simulink model "drone_diagram"  (R2021a)
settings: Solver=VariableStepAuto  StartTime=0.0  StopTime=10.0  RelTol=1e-3
values from neighbouring files (symbols this model uses):
  air_density = 1.225    [param_set.m]
  g = 9.8    [param_set.m]
  J = [Jxx 0 0; 0 Jyy 0; 0 0 Jzz]    [linearize_lqr.m]    (also in param_set.m)
  m = 1.5    [param_set.m]
  mixer_matrix = inv(dynamics_matrix)    [param_set.m]
  motor_mix_vector = [1 -1 1 -1]    [param_set.m]
  set_points = [1 0 hover_height 0 0 0 0 0 0 0 0 0]'    [linearize_lqr.m]    (also in param_set.m)
undefined symbols (not defined in the file or in its folder): c_p, lqr_K, lumped_matrix, m_b_a, motor_n_eq, offset, prop_diam, prop_j, slope, x_dist, y_dist
libraries: vrlib x3, aerolibutil x1, dspmtrx3 x1
settings Model: Creator=willwu  LastModifiedBy=Willi

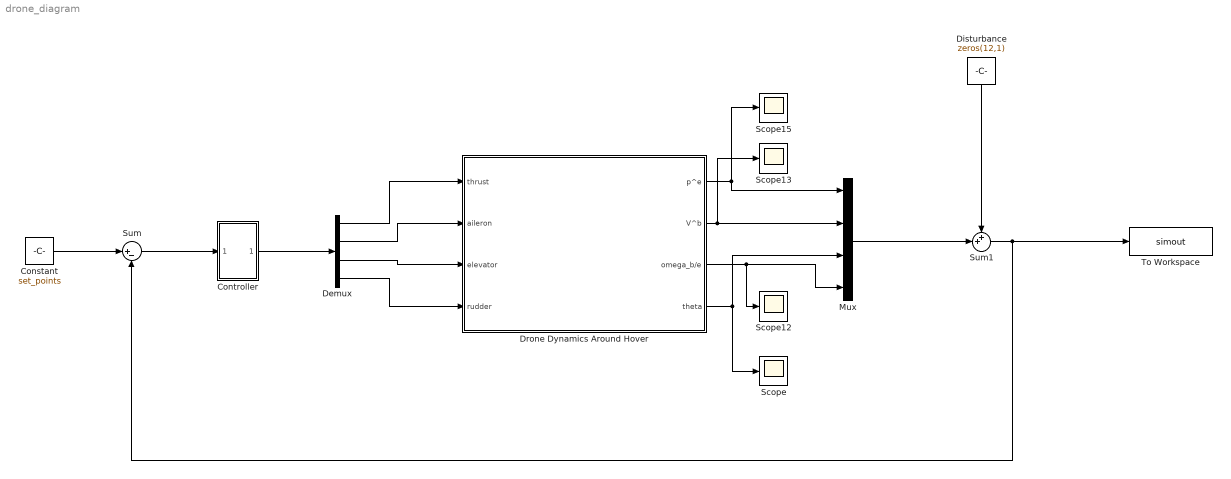
== system drone_diagram ==
  Constant : Constant  Value=set_points
  Controller : Subsystem
  Demux : Demux
  Disturbance : Constant  Value=zeros(12,1)
  Drone Dynamics Around Hover : Subsystem
  Mux : Mux
  Scope{,12..13,15} (4 alike) : Scope
  Sum : Sum  Inputs=|+-
  Sum1 : Sum  Inputs=++|
  To Workspace : ToWorkspace  VariableName=simout  SaveFormat=Timeseries  SampleTime=-1
  wires:
  Drone Dynamics Around Hover/1(p^e) -> Scope15/1, Mux/1
  Drone Dynamics Around Hover/2(V^b) -> Mux/2, Scope13/1
  Drone Dynamics Around Hover/3(omega_b/e) -> Mux/4, Scope12/1
  Drone Dynamics Around Hover/4(theta) -> Scope/1, Mux/3
  Demux/1 -> Drone Dynamics Around Hover/1(thrust)
  Demux/2 -> Drone Dynamics Around Hover/2(aileron)
  Demux/3 -> Drone Dynamics Around Hover/3(elevator)
  Demux/4 -> Drone Dynamics Around Hover/4(rudder)
  Constant/1 -> Sum/1
  Sum/1 -> Controller/1(In1)
  Controller/1(Out1) -> Demux/1
  Mux/1 -> Sum1/2
  Sum1/1 -> Sum/2, To Workspace/1
  Disturbance/1 -> Sum1/1

== system drone_diagram/Controller ==
  In1 : Inport
  Gain : Gain  Gain=lqr_K  Multiplication=Matrix(K*u)
  Out1 : Outport
  wires:
  In1/1 -> Gain/1
  Gain/1 -> Out1/1

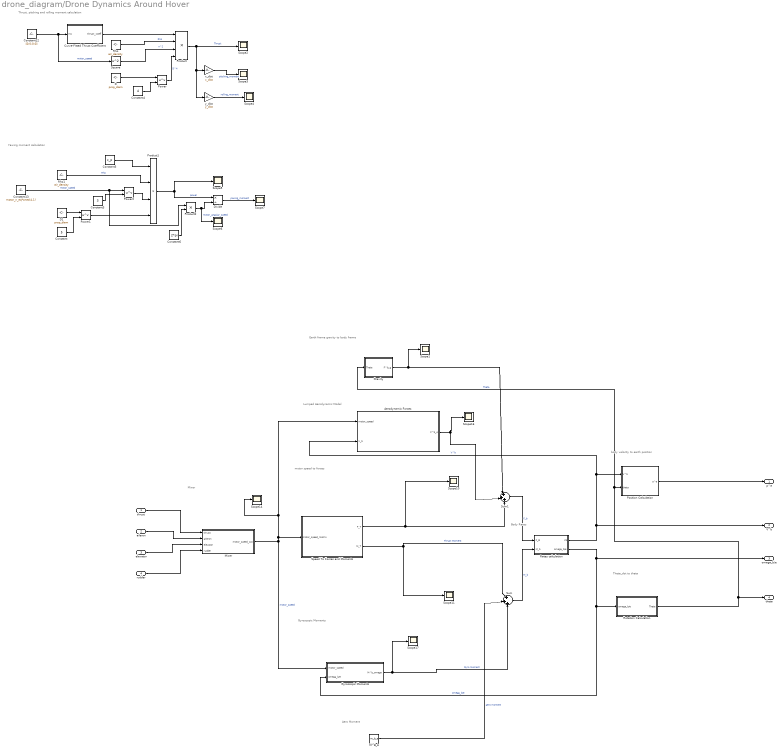
== system drone_diagram/Drone Dynamics Around Hover ==
  note: Aero Moment
  note: Mixer
  note: Gyroscopic Moments
  note: Lumped Aerodynamic Model
  note: body velocity to earth position
  note: motor speed to forces
  note: Earth frame gravity to body frame
  note: Theta_dot to theta
  note: Body Rates
  note: Yawing moment calculation
  note: Thrust, pitching and rolling moment calculation
  thrust : Inport
  aileron : Inport  Port=2
  elevator : Inport  Port=3
  rudder : Inport  Port=4
  Aerodynamic Forces : Subsystem
  Constant : Constant  Value=5
  Constant12 : Constant  Value=[0;0;0;0]
  Constant13 : Constant  Value=motor_n_eq*ones(4,1)
  Constant3 : Constant  Value=3
  Constant4 : Constant  Value=4
  Constant5 : Constant  Value=c_p
  Constant6 : Constant  Value=2*pi
  Curve-Fitted Thrust Coefficient : Subsystem
  D : Constant  Value=prop_diam
  D1 : Constant  Value=prop_diam
  Divide : Product  Inputs=*/
  Gravity : Subsystem
  Gyroscopic Moments : Subsystem
  M^B_A : Constant  Value=m_b_a
  Mixer : Subsystem
  Position Calculation : Subsystem
  Power : Math  Operator=pow  SaturateOnIntegerOverflow=on
  Power1 : Math  Operator=pow  SaturateOnIntegerOverflow=on
  Power2 : Math  Operator=pow  SaturateOnIntegerOverflow=on
  Product : Product  Inputs=4
  Product1 : Product  Inputs=4
  Product2 : Product
  Rates calculation : Subsystem
  Rho : Constant  Value=air_density
  Rho1 : Constant  Value=air_density
  Rotation Calculation : Subsystem
  Scope{1..7,10..11,14,16..17} (12 alike) : Scope
  Speed To Forces and Moments : Subsystem
  Square : Math  Operator=square  SaturateOnIntegerOverflow=on
  Sum : Sum  Inputs=|+|+|+
  Sum1 : Sum  Inputs=|+|+|+
  x_dist : Gain  Gain=x_dist
  y_dist : Gain  Gain=y_dist
  p^e : Outport
  V^b : Outport  Port=2
  omega_b/e : Outport  Port=3
  theta : Outport  Port=4
  wires:
  Sum1/1 -> Rates calculation/1(F_B)  "F_b"
  Aerodynamic Forces/1(F^b_A) -> Scope16/1, Sum1/2
  Mixer/1(motor_speed_out) -> Speed To Forces and Moments/1(motor_speed_matrix), Aerodynamic Forces/1(motor_speed), Scope14/1, Gyroscopic Moments/1(motor_speed)  "motor_speed"
  Sum/1 -> Rates calculation/2(M_b)  "M_b"
  Rotation Calculation/1(Theta) -> theta/1, Gravity/1(Theta), Position Calculation/2(theta)  "Theta"
  Rates calculation/2(omega_b/e) -> omega_b/e/1, Gyroscopic Moments/2(omega_b/e), Rotation Calculation/1(omega_b/e)  "omega_b/e"
  Speed To Forces and Moments/2(M_T) -> Sum/1, Scope11/1  "Thrust Moment"
  Gravity/1(F^b_g) -> Sum1/1, Scope1/1
  Rates calculation/1(Vb) -> V^b/1, Aerodynamic Forces/2(V_b), Position Calculation/1(V^b)  "V^b"
  Gyroscopic Moments/1(M^b_omega) -> Sum/3, Scope17/1  "Gyro moment"
  Speed To Forces and Moments/1(F_T) -> Sum1/3, Scope10/1
  M^B_A/1 -> Sum/2  "aero moment"
  Position Calculation/1(p^e) -> p^e/1
  elevator/1 -> Mixer/3(elevator)
  thrust/1 -> Mixer/1(thrust)
  aileron/1 -> Mixer/2(aileron)
  rudder/1 -> Mixer/4(rudder)
  y_dist/1 -> Scope4/1  "rolling_moment"
  Constant6/1 -> Product2/2
  Product1/1 -> Scope5/1, Divide/1  "power"
  Rho1/1 -> Product1/2  "Rho"
  Constant12/1 -> Square/1, Curve-Fitted Thrust Coefficient/1(In1)  "motor_speed"
  Power1/1 -> Product1/4
  Constant3/1 -> Power2/2
  Constant/1 -> Power1/2
  Power2/1 -> Product1/3
  D1/1 -> Power1/1
  Power/1 -> Product/4  "D^4"
  Product2/1 -> Scope6/1, Divide/2  "motor_angular_speed"
  Square/1 -> Product/3  "n^2"
  Product/1 -> Scope2/1, y_dist/1, x_dist/1  "Thrust"
  Rho/1 -> Product/2  "Rho"
  Constant4/1 -> Power/2
  Divide/1 -> Scope7/1  "yawing_moment"
  Constant5/1 -> Product1/1
  Constant13/1 -> Product2/1, Power2/1  "Motor_speed"
  x_dist/1 -> Scope3/1  "pitching_moment"
  D/1 -> Power/1
  Curve-Fitted Thrust Coefficient/1(thrust_coeff) -> Product/1

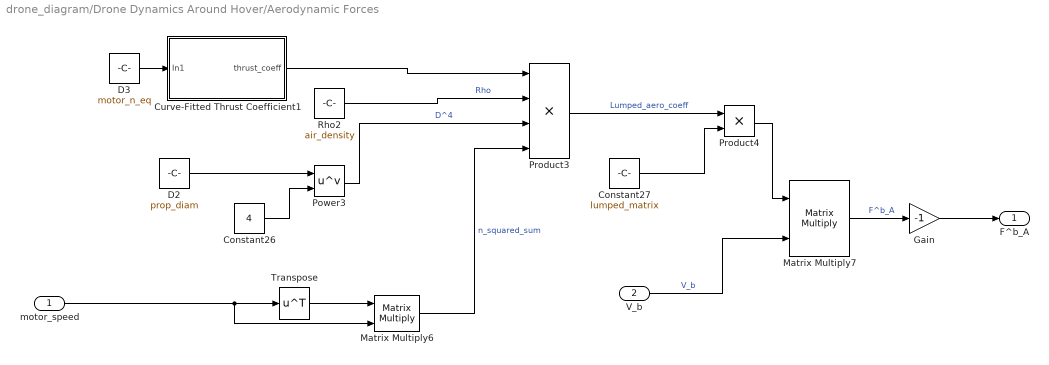
== system drone_diagram/Drone Dynamics Around Hover/Aerodynamic Forces ==
  motor_speed : Inport
  V_b : Inport  Port=2
  Constant26 : Constant  Value=4
  Constant27 : Constant  Value=lumped_matrix
  Curve-Fitted Thrust Coefficient1 : Subsystem
  D2 : Constant  Value=prop_diam
  D3 : Constant  Value=motor_n_eq
  Gain : Gain  Gain=-1
  Matrix Multiply6 : Product  Multiplication=Matrix(*)
  Matrix Multiply7 : Product  Multiplication=Matrix(*)
  Power3 : Math  Operator=pow  SaturateOnIntegerOverflow=on
  Product3 : Product  Inputs=4
  Product4 : Product
  Rho2 : Constant  Value=air_density
  Transpose : Math  Operator=transpose  SaturateOnIntegerOverflow=on
  F^b_A : Outport
  wires:
  V_b/1 -> Matrix Multiply7/2  "V_b"
  Matrix Multiply6/1 -> Product3/4  "n_squared_sum"
  Power3/1 -> Product3/3  "D^4"
  D3/1 -> Curve-Fitted Thrust Coefficient1/1(In1)
  Constant27/1 -> Product4/2
  Rho2/1 -> Product3/2  "Rho"
  Product3/1 -> Product4/1  "Lumped_aero_coeff"
  motor_speed/1 -> Matrix Multiply6/2, Transpose/1
  Product4/1 -> Matrix Multiply7/1
  Transpose/1 -> Matrix Multiply6/1
  Constant26/1 -> Power3/2
  D2/1 -> Power3/1
  Curve-Fitted Thrust Coefficient1/1(thrust_coeff) -> Product3/1
  Matrix Multiply7/1 -> Gain/1  "F^b_A"
  Gain/1 -> F^b_A/1

== system drone_diagram/Drone Dynamics Around Hover/Curve-Fitted Thrust Coefficient ==
  In1 : Inport
  Constant : Constant  Value=offset
  Gain2 : Gain  Gain=slope
  Sum2 : Sum  Inputs=|++
  thrust_coeff : Outport
  wires:
  Constant/1 -> Sum2/2  "offset"
  Gain2/1 -> Sum2/1  "slope * n"
  Sum2/1 -> thrust_coeff/1  "thrust_coeff"
  In1/1 -> Gain2/1

== system drone_diagram/Drone Dynamics Around Hover/Gravity ==
  Theta : Inport
  Constant11 : Constant  Value=[0;0;-m*g]
  Matrix Multiply3 : Product  Multiplication=Matrix(*)
  theta_2_rotate E->b : MATLAB Function  TreatAsAtomicUnit=on
  F^b_g : Outport
  wires:
  theta_2_rotate E->b/1(y) -> Matrix Multiply3/1  "RE->b"
  Constant11/1 -> Matrix Multiply3/2  "F^e_g"
  Matrix Multiply3/1 -> F^b_g/1  "F^b_g"
  Theta/1 -> theta_2_rotate E->b/1(u)

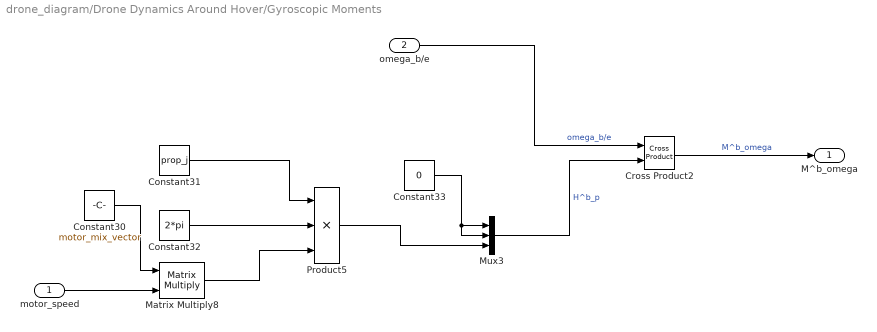
== system drone_diagram/Drone Dynamics Around Hover/Gyroscopic Moments ==
  motor_speed : Inport
  omega_b/e : Inport  Port=2
  Constant30 : Constant  Value=motor_mix_vector  VectorParams1D=off
  Constant31 : Constant  Value=prop_j
  Constant32 : Constant  Value=2*pi
  Constant33 : Constant  Value=0
  Cross Product2 : vrlib/Utilities/Cross Product
  Matrix Multiply8 : Product  Multiplication=Matrix(*)
  Mux3 : Mux  Inputs=3
  Product5 : Product  Inputs=3
  M^b_omega : Outport
  wires:
  Constant30/1 -> Matrix Multiply8/1
  Constant33/1 -> Mux3/2, Mux3/1
  Matrix Multiply8/1 -> Product5/3
  Constant32/1 -> Product5/2
  Product5/1 -> Mux3/3
  omega_b/e/1 -> Cross Product2/1  "omega_b/e"
  Constant31/1 -> Product5/1
  Mux3/1 -> Cross Product2/2  "H^b_p"
  motor_speed/1 -> Matrix Multiply8/2
  Cross Product2/1 -> M^b_omega/1  "M^b_omega"

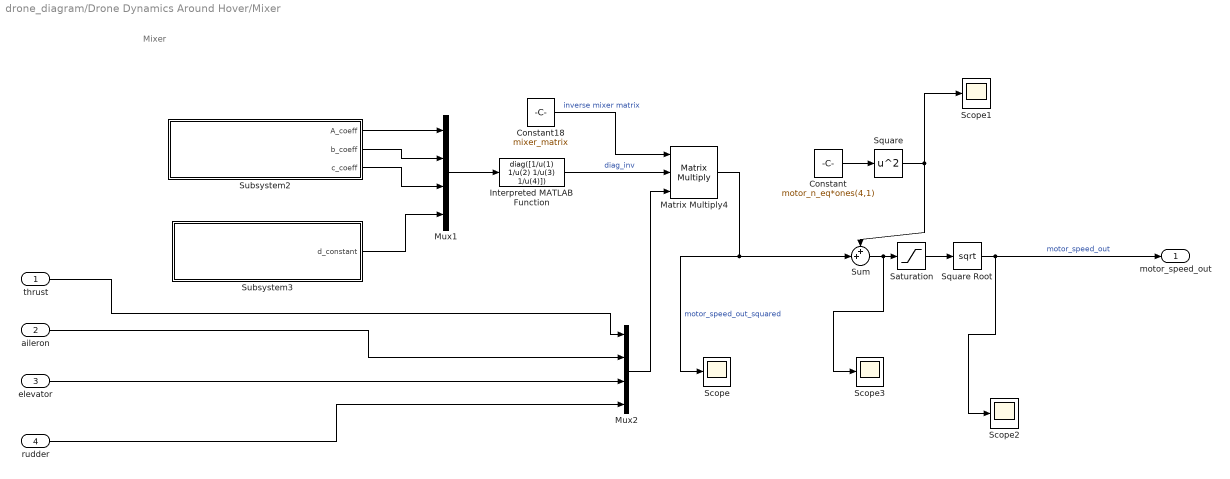
== system drone_diagram/Drone Dynamics Around Hover/Mixer ==
  note: Mixer
  thrust : Inport
  aileron : Inport  Port=2
  elevator : Inport  Port=3
  rudder : Inport  Port=4
  Constant : Constant  Value=motor_n_eq*ones(4,1)
  Constant18 : Constant  Value=mixer_matrix
  Interpreted MATLAB Function : MATLABFcn  MATLABFcn=diag([1/u(1) 1/u(2) 1/u(3) 1/u(4)])  OutputDimensions=[4 4]  Output1D=off
  Matrix Multiply4 : Product  Inputs=3  Multiplication=Matrix(*)
  Mux1 : Mux
  Mux2 : Mux
  Saturation : Saturate  UpperLimit=inf  LowerLimit=0
  Scope{,1..3} (4 alike) : Scope
  Square : Math  Operator=square  SaturateOnIntegerOverflow=on
  Square Root : Sqrt  SaturateOnIntegerOverflow=on
  Subsystem2 : Subsystem
  Subsystem3 : Subsystem
  Sum : Sum  Inputs=++|
  motor_speed_out : Outport
  wires:
  Subsystem2/1(A_coeff) -> Mux1/1
  Subsystem3/1(d_constant) -> Mux1/4
  Subsystem2/2(b_coeff) -> Mux1/2
  Mux1/1 -> Interpreted MATLAB Function/1
  Constant18/1 -> Matrix Multiply4/1  "inverse mixer matrix"
  rudder/1 -> Mux2/4
  Subsystem2/3(c_coeff) -> Mux1/3
  Interpreted MATLAB Function/1 -> Matrix Multiply4/2  "diag_inv"
  Mux2/1 -> Matrix Multiply4/3
  Matrix Multiply4/1 -> Sum/2, Scope/1  "motor_speed_out_squared"
  aileron/1 -> Mux2/2
  thrust/1 -> Mux2/1
  elevator/1 -> Mux2/3
  Constant/1 -> Square/1
  Square/1 -> Sum/1, Scope1/1
  Square Root/1 -> Scope2/1, motor_speed_out/1  "motor_speed_out"
  Sum/1 -> Scope3/1, Saturation/1
  Saturation/1 -> Square Root/1

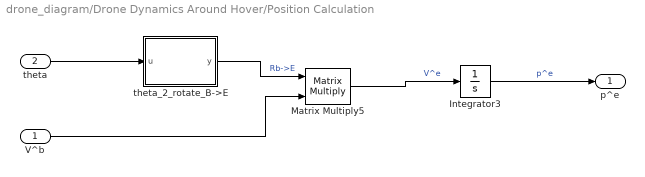
== system drone_diagram/Drone Dynamics Around Hover/Position Calculation ==
  V^b : Inport
  theta : Inport  Port=2
  Integrator3 : Integrator
  Matrix Multiply5 : Product  Multiplication=Matrix(*)
  theta_2_rotate_B->E : MATLAB Function  TreatAsAtomicUnit=on
  p^e : Outport
  wires:
  Matrix Multiply5/1 -> Integrator3/1  "V^e"
  theta/1 -> theta_2_rotate_B->E/1(u)
  theta_2_rotate_B->E/1(y) -> Matrix Multiply5/1  "Rb->E"
  Integrator3/1 -> p^e/1  "p^e"
  V^b/1 -> Matrix Multiply5/2

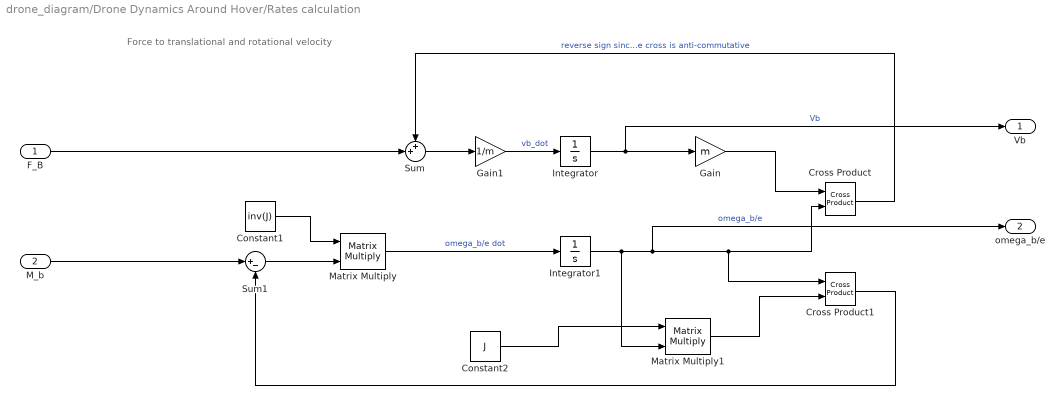
== system drone_diagram/Drone Dynamics Around Hover/Rates calculation ==
  note: Force to translational and rotational velocity
  F_B : Inport
  M_b : Inport  Port=2
  Constant1 : Constant  Value=inv(J)
  Constant2 : Constant  Value=J
  Cross Product : vrlib/Utilities/Cross Product
  Cross Product1 : vrlib/Utilities/Cross Product
  Gain : Gain  Gain=m
  Gain1 : Gain  Gain=1/m
  Integrator : Integrator
  Integrator1 : Integrator
  Matrix Multiply : Product  Multiplication=Matrix(*)
  Matrix Multiply1 : Product  Multiplication=Matrix(*)
  Sum : Sum  Inputs=++|
  Sum1 : Sum  Inputs=|+-
  Vb : Outport
  omega_b/e : Outport  Port=2
  wires:
  F_B/1 -> Sum/2
  M_b/1 -> Sum1/1
  Gain1/1 -> Integrator/1  "vb_dot"
  Sum1/1 -> Matrix Multiply/2
  Sum/1 -> Gain1/1
  Cross Product/1 -> Sum/1  "reverse sign since cross is anti-commutative"
  Matrix Multiply/1 -> Integrator1/1  "omega_b/e dot"
  Gain/1 -> Cross Product/1
  Cross Product1/1 -> Sum1/2
  Integrator/1 -> Gain/1, Vb/1  "Vb"
  Constant1/1 -> Matrix Multiply/1
  Integrator1/1 -> Cross Product1/1, Cross Product/2, omega_b/e/1, Matrix Multiply1/2  "omega_b/e"
  Matrix Multiply1/1 -> Cross Product1/2
  Constant2/1 -> Matrix Multiply1/1

== system drone_diagram/Drone Dynamics Around Hover/Rotation Calculation ==
  omega_b/e : Inport
  H : MATLABFcn  MATLABFcn=[1 0 -sin(u(2)); 0 cos(u(1)) sin(u(1))*cos(u(2)); 0 -sin(u(1)) cos(u(1))*cos(u(2))]  OutputDimensions=[3 3]  Output1D=off
  Integrator2 : Integrator
  Invert 3x3 Matrix : aerolibutil/Invert  3x3 Matrix
  Matrix Multiply2 : Product  Multiplication=Matrix(*)
  Theta : Outport
  wires:
  Integrator2/1 -> Theta/1, H/1  "Theta"
  Matrix Multiply2/1 -> Integrator2/1  "Theta_dot"
  H/1 -> Invert 3x3 Matrix/1  "H"
  omega_b/e/1 -> Matrix Multiply2/2
  Invert 3x3 Matrix/1 -> Matrix Multiply2/1  "H_inv"

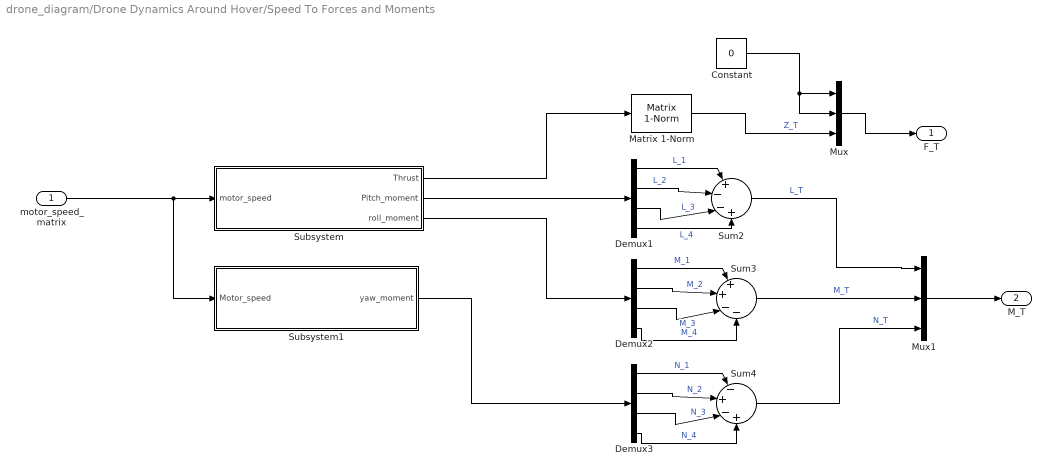
== system drone_diagram/Drone Dynamics Around Hover/Speed To Forces and Moments ==
  motor_speed_matrix : Inport
  Constant : Constant  Value=0
  Demux1 : Demux
  Demux2 : Demux
  Demux3 : Demux
  Matrix 1-Norm : dspmtrx3/Matrix  1-Norm  roundingMode=Floor  overflowMode=off  outputDataTypeStr=Inherit: Same as accumulator  outputMin=[]  outputMax=[]  outputLastDataTypeStr=Inherit: Same as accumulator
      settings: SourceProductBaseCode=DS
  Mux : Mux  Inputs=3
  Mux1 : Mux  Inputs=3
  Subsystem : Subsystem
  Subsystem1 : Subsystem
  Sum2 : Sum  Inputs=|+|-|-|+
  Sum3 : Sum  Inputs=|+|+|-|-
  Sum4 : Sum  Inputs=|-|+|-|+
  F_T : Outport
  M_T : Outport  Port=2
  wires:
  Demux1/1 -> Sum2/1  "L_1"
  Demux3/1 -> Sum4/1  "N_1"
  Subsystem/1(Thrust) -> Matrix 1-Norm/1
  Demux1/3 -> Sum2/3  "L_3"
  Demux3/4 -> Sum4/4  "N_4"
  motor_speed_matrix/1 -> Subsystem1/1(Motor_speed), Subsystem/1(motor_speed)
  Demux2/1 -> Sum3/1  "M_1"
  Sum4/1 -> Mux1/3  "N_T"
  Demux3/3 -> Sum4/3  "N_3"
  Demux2/4 -> Sum3/4  "M_4"
  Demux3/2 -> Sum4/2  "N_2"
  Demux2/3 -> Sum3/3  "M_3"
  Demux1/2 -> Sum2/2  "L_2"
  Subsystem/3(roll_moment) -> Demux2/1
  Demux1/4 -> Sum2/4  "L_4"
  Demux2/2 -> Sum3/2  "M_2"
  Subsystem1/1(yaw_moment) -> Demux3/1
  Subsystem/2(Pitch_moment) -> Demux1/1
  Sum3/1 -> Mux1/2  "M_T"
  Matrix 1-Norm/1 -> Mux/3  "Z_T"
  Constant/1 -> Mux/2, Mux/1
  Mux/1 -> F_T/1
  Mux1/1 -> M_T/1
  Sum2/1 -> Mux1/1  "L_T"

== system drone_diagram/Drone Dynamics Around Hover/Aerodynamic Forces/Curve-Fitted Thrust Coefficient1 ==
  In1 : Inport
  Constant : Constant  Value=offset
  Gain2 : Gain  Gain=slope
  Sum2 : Sum  Inputs=|++
  thrust_coeff : Outport
  wires:
  In1/1 -> Gain2/1
  Sum2/1 -> thrust_coeff/1  "thrust_coeff"
  Gain2/1 -> Sum2/1  "slope * n"
  Constant/1 -> Sum2/2  "offset"

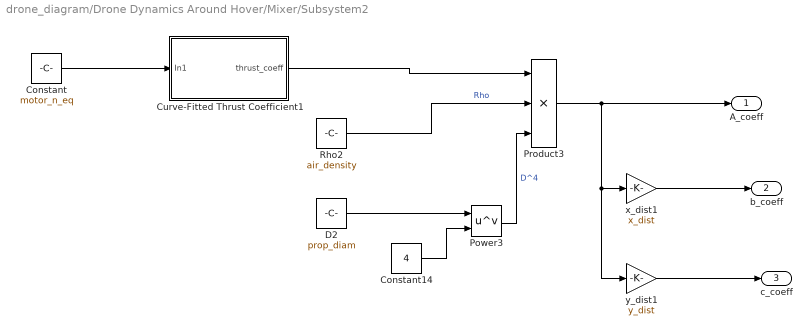
== system drone_diagram/Drone Dynamics Around Hover/Mixer/Subsystem2 ==
  Constant : Constant  Value=motor_n_eq
  Constant14 : Constant  Value=4
  Curve-Fitted Thrust Coefficient1 : Subsystem
  D2 : Constant  Value=prop_diam
  Power3 : Math  Operator=pow  SaturateOnIntegerOverflow=on
  Product3 : Product  Inputs=3
  Rho2 : Constant  Value=air_density
  x_dist1 : Gain  Gain=x_dist
  y_dist1 : Gain  Gain=y_dist
  A_coeff : Outport
  b_coeff : Outport  Port=2
  c_coeff : Outport  Port=3
  wires:
  y_dist1/1 -> c_coeff/1
  x_dist1/1 -> b_coeff/1
  Curve-Fitted Thrust Coefficient1/1(thrust_coeff) -> Product3/1
  Constant/1 -> Curve-Fitted Thrust Coefficient1/1(In1)
  D2/1 -> Power3/1
  Constant14/1 -> Power3/2
  Rho2/1 -> Product3/2  "Rho"
  Product3/1 -> A_coeff/1, y_dist1/1, x_dist1/1
  Power3/1 -> Product3/3  "D^4"

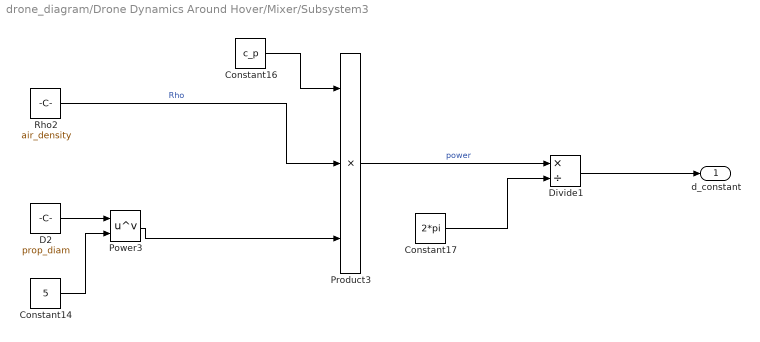
== system drone_diagram/Drone Dynamics Around Hover/Mixer/Subsystem3 ==
  Constant14 : Constant  Value=5
  Constant16 : Constant  Value=c_p
  Constant17 : Constant  Value=2*pi
  D2 : Constant  Value=prop_diam
  Divide1 : Product  Inputs=*/
  Power3 : Math  Operator=pow  SaturateOnIntegerOverflow=on
  Product3 : Product  Inputs=3
  Rho2 : Constant  Value=air_density
  d_constant : Outport
  wires:
  Divide1/1 -> d_constant/1
  Rho2/1 -> Product3/2  "Rho"
  D2/1 -> Power3/1
  Constant16/1 -> Product3/1
  Power3/1 -> Product3/3
  Constant14/1 -> Power3/2
  Constant17/1 -> Divide1/2
  Product3/1 -> Divide1/1  "power"

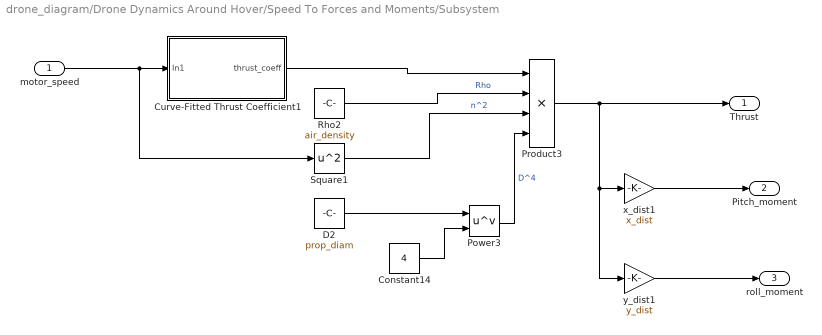
== system drone_diagram/Drone Dynamics Around Hover/Speed To Forces and Moments/Subsystem ==
  motor_speed : Inport
  Constant14 : Constant  Value=4
  Curve-Fitted Thrust Coefficient1 : Subsystem
  D2 : Constant  Value=prop_diam
  Power3 : Math  Operator=pow  SaturateOnIntegerOverflow=on
  Product3 : Product  Inputs=4
  Rho2 : Constant  Value=air_density
  Square1 : Math  Operator=square  SaturateOnIntegerOverflow=on
  x_dist1 : Gain  Gain=x_dist
  y_dist1 : Gain  Gain=y_dist
  Thrust : Outport
  Pitch_moment : Outport  Port=2
  roll_moment : Outport  Port=3
  wires:
  Power3/1 -> Product3/4  "D^4"
  Product3/1 -> x_dist1/1, y_dist1/1, Thrust/1
  Rho2/1 -> Product3/2  "Rho"
  Constant14/1 -> Power3/2
  D2/1 -> Power3/1
  motor_speed/1 -> Curve-Fitted Thrust Coefficient1/1(In1), Square1/1
  Square1/1 -> Product3/3  "n^2"
  Curve-Fitted Thrust Coefficient1/1(thrust_coeff) -> Product3/1
  x_dist1/1 -> Pitch_moment/1
  y_dist1/1 -> roll_moment/1

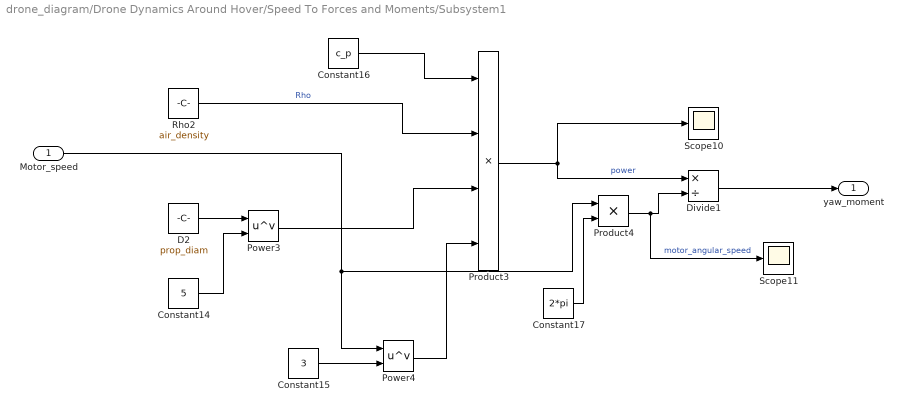
== system drone_diagram/Drone Dynamics Around Hover/Speed To Forces and Moments/Subsystem1 ==
  Motor_speed : Inport
  Constant14 : Constant  Value=5
  Constant15 : Constant  Value=3
  Constant16 : Constant  Value=c_p
  Constant17 : Constant  Value=2*pi
  D2 : Constant  Value=prop_diam
  Divide1 : Product  Inputs=*/
  Power3 : Math  Operator=pow  SaturateOnIntegerOverflow=on
  Power4 : Math  Operator=pow  SaturateOnIntegerOverflow=on
  Product3 : Product  Inputs=4
  Product4 : Product
  Rho2 : Constant  Value=air_density
  Scope10 : Scope
  Scope11 : Scope
  yaw_moment : Outport
  wires:
  Product3/1 -> Scope10/1, Divide1/1  "power"
  Product4/1 -> Divide1/2, Scope11/1  "motor_angular_speed"
  Constant14/1 -> Power3/2
  Constant17/1 -> Product4/2
  Power4/1 -> Product3/4
  Motor_speed/1 -> Power4/1, Product4/1
  Power3/1 -> Product3/3
  Constant16/1 -> Product3/1
  Constant15/1 -> Power4/2
  D2/1 -> Power3/1
  Rho2/1 -> Product3/2  "Rho"
  Divide1/1 -> yaw_moment/1

== system drone_diagram/Drone Dynamics Around Hover/Mixer/Subsystem2/Curve-Fitted Thrust Coefficient1 ==
  In1 : Inport
  Constant : Constant  Value=offset
  Gain2 : Gain  Gain=slope
  Sum2 : Sum  Inputs=|++
  thrust_coeff : Outport
  wires:
  Constant/1 -> Sum2/2  "offset"
  Gain2/1 -> Sum2/1  "slope * n"
  Sum2/1 -> thrust_coeff/1  "thrust_coeff"
  In1/1 -> Gain2/1

== system drone_diagram/Drone Dynamics Around Hover/Speed To Forces and Moments/Subsystem/Curve-Fitted Thrust Coefficient1 ==
  In1 : Inport
  Constant : Constant  Value=offset
  Gain2 : Gain  Gain=slope
  Sum2 : Sum  Inputs=|++
  thrust_coeff : Outport
  wires:
  In1/1 -> Gain2/1
  Sum2/1 -> thrust_coeff/1  "thrust_coeff"
  Gain2/1 -> Sum2/1  "slope * n"
  Constant/1 -> Sum2/2  "offset"

== matlab function drone_diagram/Drone Dynamics Around Hover/Gravity/theta_2_rotate E->b ==
  data: u input; y output
function y = fcn(u)
    phi = u(1);
    theta = u(2);
    psi = u(3);
    
    R_phi = [1 0 0;0 cos(phi) sin(phi); 0 -sin(phi) cos(phi)];
    R_theta = [cos(theta) 0 -sin(theta); 0 1 0; sin(theta) 0 cos(theta)];
    R_psi = [cos(psi) sin(psi) 0; -sin(psi) cos(psi) 0; 0 0 1];
    
y = R_phi * R_theta * R_psi;

== matlab function drone_diagram/Drone Dynamics Around Hover/Position Calculation/theta_2_rotate_B->E ==
  data: u input; y output
function y = fcn(u)
    phi = u(1);
    theta = u(2);
    psi = u(3);
    
    R_phi = [1 0 0;0 cos(phi) sin(phi); 0 -sin(phi) cos(phi)];
    R_theta = [cos(theta) 0 -sin(theta); 0 1 0; sin(theta) 0 cos(theta)];
    R_psi = [cos(psi) sin(psi) 0; -sin(psi) cos(psi) 0; 0 0 1];
    
y =  R_psi' * R_theta' * R_phi';
